simulink model "rotpentemplate"  (R2021b)
settings: Solver=ode45  StartTime=0.0  StopTime=10  RelTol=1e-3  EnableMultiTasking=on
values from neighbouring files (symbols this model uses):
  A = [0 1 0 0 ... (first row only)    [linearize_script.m]    (also in step4_0_linearize_operating_point.m = double(A); step4_linearized_system.mat = [0 0.306815158551 0 -109.913929424 0 1 -60.0152130057 0 126.; syms_test.m = double(A))
  adingain = [adin_gain 1 1 1 1 1]    [hwinit.m]    (also in hwinit_raw.m)
  adinoffs = [adin_offs 0 0 0 0 0]    [hwinit.m]    (also in hwinit_raw.m)
  B = [0 ... (first row only)    [linearize_script.m]    (also in step4_0_linearize_operating_point.m = double(B); step4_linearized_system.mat = [0 0 0 0 858.38566108]; syms_test.m = double(B))
  C = [1 0 0 0 ... (first row only)    [linearize_script.m]    (also in matrixmaker_linearization.m = [b_1_0 - P_3 * theta_d_2 * sin(theta_2)  -P_3 * (theta_d_1 +; step4_0_linearize_operating_point.m = [1 0 0 0 0; step4_linearized_system.mat = [1  0  0  0  0; 0  0  1  0  0]; syms_test.m)
  D = zeros(2,1)    [linearize_script.m]    (also in step4_0_linearize_operating_point.m; step4_linearized_system.mat = [0 0]; syms_test.m)
  daoutgain = 1*[-6]    [hwinit.m]    (also in hwinit_raw.m)
  daoutoffs = [0.00]    [hwinit.m]    (also in hwinit_raw.m)
  h = 0.001    [hwinit.m]    (also in hwinit_raw.m; init_fugi.m = fugiboard('Open', 'Pendulum1'); one_run.m = fugiboard('Open', 'pendulum1'); one_single_run.m = fugiboard('Open', 'pendulum1'))
  K = K1    [step6_1_controller_feedback.m]
  Ke = [165.387583111  -5.89857635124; 3165.93278733  -398.274578992; 81.102554045  215.74157361; 15046.5760039  11054.3649817; 3886.10400765  -704.144825536]    [step5_observor.mat]    (also in step5_observor_design.m = place(A_, B_, 0.5*J)')
  theta_1_0 = pi    (= 3.14159265359)    [hwinit.m]    (also in hwinit_raw.m; step4_0_linearize_operating_point.m; step5_observor_design.m = x_op(1); step6_1_controller_feedback.m = x_op(1))
  theta_2_0 = 0    [hwinit.m]    (also in hwinit_raw.m; step4_0_linearize_operating_point.m; step5_observor_design.m = x_op(3); step6_1_controller_feedback.m = x_op(3))
libraries: slpidlib x2
settings Model: Creator=rbabuska  LastModifiedBy=lyitingli
settings SolverCC: AlgebraicLoopSolver=TrustRegion
settings DataIOCC: LimitDataPoints=on  SaveFormat=Array  ReturnWorkspaceOutputs=off  SignalLoggingName=sigsOut
settings OptimizationCC: BooleanDataType=off  ExpressionDepthLimit=2147483647  InitFltsAndDblsToZero=on  LifeSpan=inf
settings DebuggingCC: SaveWithParameterizedLinksMsg=none  SignalResolutionControl=TryResolveAllWithWarning  MultiTaskDSMMsg=warning  MultiTaskCondExecSysMsg=none  AllowSymbolicDim=off  StateNameClashWarn=warning  SFUnexpectedBacktrackingDiag=warning  SFNoUnconditionalDefaultTransitionDiag=warning  SFExecutionAtInitializationDiag=none  SFMachineParentedDataDiag=warning  ArithmeticOperatorsInVariantConditions=warning
settings HardwareCC: ProdBitPerPointer=32  ProdBitPerSizeT=32  ProdBitPerPtrDiffT=32  ProdLargestAtomicFloat=None  ProdIntDivRoundTo=Undefined  ProdEndianess=Unspecified  ProdWordSize=32  ProdHWDeviceType=32-bit Generic  TargetUnknown=on
settings ModelReferenceCC: PropagateSignalLabelsOutOfModel=off
settings SFSimCC: SimUseLocalCustomCode=off  CustomCodeUndefinedFunction=UseInterfaceOnly
settings RTWCC: RTWUseLocalCustomCode=off
settings CodeAppCC: StateflowObjectComments=on
settings GRTTargetCC: TargetFcnLib=ansi_tfl_tmw.mat  TargetLangStandard=C89/C90 (ANSI)  CombineOutputUpdateFcns=off  GRTInterface=on
settings ConfigComp: CovMetricSettings=dw  CovSaveCumulativeToWorkspaceVar=on  CovSaveSingleToWorkspaceVar=on  CovExternalEMLEnable=off

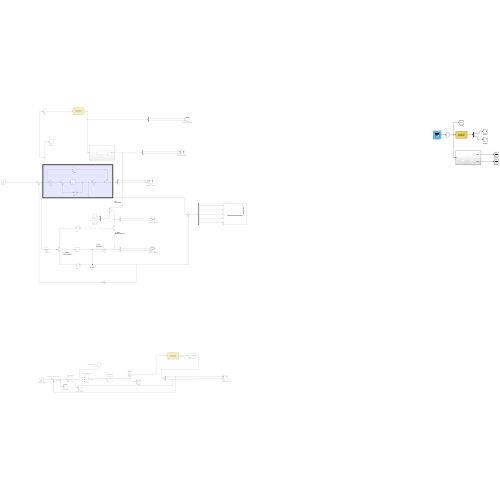
[thumbnail: Simulink's stored preview of the top-level diagram]
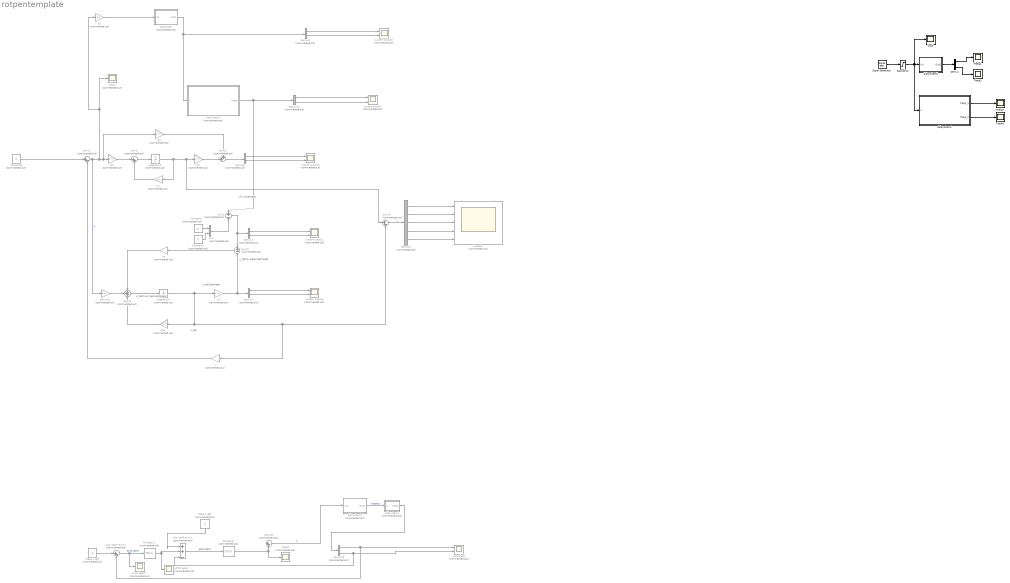
== system rotpentemplate ==
  note: y_hat(k)
      | output estimate
  note: x_hat(k+1)
      | next estimate
  note: y(k)
      | incremetal
  note: x_hat
      | Estimate
  note: x_hat
  A2 : Gain  Commented=on  Gain=A  Multiplication=Matrix(K*u) (u vector)
  B1 : Gain  Commented=on  Gain=-0.1
  B4 : Gain  Commented=on  Gain=B  Multiplication=Matrix(K*u)
  B5 : Gain  Commented=on  Gain=D  Multiplication=Matrix(K*u)
  C3 : Gain  Commented=on  Gain=C  Multiplication=Matrix(K*u) (u vector)
  C4 : Gain  Commented=on  Gain=C  Multiplication=Matrix(K*u) (u vector)
  Constant1 : Constant  Commented=on  Value=pi  SampleTime=-1
  Constant2 : Constant  Commented=on  Value=0  SampleTime=-1
  Constant3 : Constant  Commented=on  Value=0  SampleTime=0.001
  Demux : Demux  Outputs=2
  Demux{1..2,5,7,11,15} (6 alike) : Demux  Commented=on  Outputs=2
  Demux6 : Demux  Commented=on  Outputs=5
  Input : Scope
  Integrator3 : Integrator  Commented=on  InitialCondition=[0; 0; 0; 0; 0]
  Integrator4 : Integrator  Commented=on  InitialCondition=[0; 0; 0; 0; 0]
  Ke : Gain  Commented=on  Gain=Ke  Multiplication=Matrix(K*u) (u vector)
  L : Gain  Commented=on  Gain=1*K  Multiplication=Matrix(K*u) (u vector)
  Mux : Mux  Commented=on  Inputs=2
  PID beam1 : slpidlib/PID Controller  Commented=on  Controller=PID  Form=Parallel  TimeDomain=Continuous-time  UseExternalTs=off  SampleTime=-1  IntegratorMethod=Forward Euler  FilterMethod=Forward Euler  ControllerParametersSource=internal  P=-0.5  I=0  D=-0.02  UseFilter=on  N=100  TunerSelectOption=Transfer Function Based (PID Tuner App)  InitialConditionSource=internal  InitialConditionForIntegrator=0  InitialConditionForFilter=0  DifferentiatorICPrevScaledInput=0  ExternalReset=none  TrackingMode=off  Kt=1  LimitOutput=off  SatLimitsSource=internal  UpperSaturationLimit=inf  LowerSaturationLimit=-inf  LinearizeAsGain=on  AntiWindupMode=none  Kb=1  POutMin=[]  POutMax=[]  IOutMin=[]  IOutMax=[]  DOutMin=[]  DOutMax=[]  NOutMin=[]  NOutMax=[]  SumOutMin=[]  SumOutMax=[]  SaturationOutMin=[]  SaturationOutMax=[]  PParamMin=[]  PParamMax=[]  IParamMin=[]  IParamMax=[]  DParamMin=[]  DParamMax=[]  NParamMin=[]  NParamMax=[]  KbParamMin=[]  KbParamMax=[]  KtParamMin=[]  KtParamMax=[]  KbOutMin=[]  KbOutMax=[]  KtOutMin=[]  KtOutMax=[]  IntegratorOutMin=[]  IntegratorOutMax=[]  FilterOutMin=[]  FilterOutMax=[]  SumI1OutMin=[]  SumI1OutMax=[]  SumI2OutMin=[]  SumI2OutMax=[]  SumI3OutMin=[]  SumI3OutMax=[]  SumI4OutMin=[]  SumI4OutMax=[]  SumDOutMin=[]  SumDOutMax=[]  DifferentiatorOutMin=[]  DifferentiatorOutMax=[]  FilterDiffOutCoefMin=[]  FilterDiffOutCoefMax=[]  ReciprocalOutMin=[]  ReciprocalOutMax=[]  SumDenOutMin=[]  SumDenOutMax=[]  SumNumOutMin=[]  SumNumOutMax=[]  DivideOutMin=[]  DivideOutMax=[]  UdiffTsProdOutMin=[]  UdiffTsProdOutMax=[]  NTsProdOutMin=[]  NTsProdOutMax=[]  UintegralTsProdOutMin=[]  UintegralTsProdOutMax=[]  UngainTsProdOutMin=[]  UngainTsProdOutMax=[]  IntegratorContinuousStateAttributes=''  IntegratorStateMustResolveToSignalObject=off  IntegratorRTWStateStorageClass=Auto  FilterContinuousStateAttributes=''  FilterStateMustResolveToSignalObject=off  FilterRTWStateStorageClass=Auto  ParallelPVariant=InternalParameters  IdealPVariant=Disabled  IVariant=InternalParameters  DVariant=InternalParameters  IntegratorVariant=Continuous  SatVariant=Disabled  AWVariant=Passthrough  PCopyVariant=Disabled  TRVariant=Disabled  FdbkBlocksVariant=Forward  IdealPFdbkVariant=Disabled  SatFdbkVariant=Disabled  DerivativeFilterVariant=ContFilter  NVariant=InternalParameters  NCopyVariant=Disabled  FilterICVariant=InternalICsFilter  IntegratorICVariant=InternalICs  ExternalResetVariant=Disabled  TRSumVariant=Passthrough  SumFdbkVariant=Disabled  SumVariant=Sum_PID  TsampFilterVariant=InternalTs  TsampNgainVariant=Passthrough  TsampIntegralVariant=Passthrough  ExternalSaturationOutDataTypeStr=Inherit: Same as second input
  PID pend1 : slpidlib/PID Controller  Commented=on  Controller=PID  Form=Parallel  TimeDomain=Continuous-time  UseExternalTs=off  SampleTime=-1  IntegratorMethod=Forward Euler  FilterMethod=Forward Euler  ControllerParametersSource=internal  P=-10  I=0  D=-0.01  UseFilter=on  N=100  TunerSelectOption=Transfer Function Based (PID Tuner App)  InitialConditionSource=internal  InitialConditionForIntegrator=0  InitialConditionForFilter=0  DifferentiatorICPrevScaledInput=0  ExternalReset=none  TrackingMode=off  Kt=1  LimitOutput=off  SatLimitsSource=internal  UpperSaturationLimit=inf  LowerSaturationLimit=-inf  LinearizeAsGain=on  AntiWindupMode=none  Kb=1  POutMin=[]  POutMax=[]  IOutMin=[]  IOutMax=[]  DOutMin=[]  DOutMax=[]  NOutMin=[]  NOutMax=[]  SumOutMin=[]  SumOutMax=[]  SaturationOutMin=[]  SaturationOutMax=[]  PParamMin=[]  PParamMax=[]  IParamMin=[]  IParamMax=[]  DParamMin=[]  DParamMax=[]  NParamMin=[]  NParamMax=[]  KbParamMin=[]  KbParamMax=[]  KtParamMin=[]  KtParamMax=[]  KbOutMin=[]  KbOutMax=[]  KtOutMin=[]  KtOutMax=[]  IntegratorOutMin=[]  IntegratorOutMax=[]  FilterOutMin=[]  FilterOutMax=[]  SumI1OutMin=[]  SumI1OutMax=[]  SumI2OutMin=[]  SumI2OutMax=[]  SumI3OutMin=[]  SumI3OutMax=[]  SumI4OutMin=[]  SumI4OutMax=[]  SumDOutMin=[]  SumDOutMax=[]  DifferentiatorOutMin=[]  DifferentiatorOutMax=[]  FilterDiffOutCoefMin=[]  FilterDiffOutCoefMax=[]  ReciprocalOutMin=[]  ReciprocalOutMax=[]  SumDenOutMin=[]  SumDenOutMax=[]  SumNumOutMin=[]  SumNumOutMax=[]  DivideOutMin=[]  DivideOutMax=[]  UdiffTsProdOutMin=[]  UdiffTsProdOutMax=[]  NTsProdOutMin=[]  NTsProdOutMax=[]  UintegralTsProdOutMin=[]  UintegralTsProdOutMax=[]  UngainTsProdOutMin=[]  UngainTsProdOutMax=[]  IntegratorContinuousStateAttributes=''  IntegratorStateMustResolveToSignalObject=off  IntegratorRTWStateStorageClass=Auto  FilterContinuousStateAttributes=''  FilterStateMustResolveToSignalObject=off  FilterRTWStateStorageClass=Auto  ParallelPVariant=InternalParameters  IdealPVariant=Disabled  IVariant=InternalParameters  DVariant=InternalParameters  IntegratorVariant=Continuous  SatVariant=Disabled  AWVariant=Passthrough  PCopyVariant=Disabled  TRVariant=Disabled  FdbkBlocksVariant=Forward  IdealPFdbkVariant=Disabled  SatFdbkVariant=Disabled  DerivativeFilterVariant=ContFilter  NVariant=InternalParameters  NCopyVariant=Disabled  FilterICVariant=InternalICsFilter  IntegratorICVariant=InternalICs  ExternalResetVariant=Disabled  TRSumVariant=Passthrough  SumFdbkVariant=Disabled  SumVariant=Sum_PID  TsampFilterVariant=InternalTs  TsampNgainVariant=Passthrough  TsampIntegralVariant=Passthrough  ExternalSaturationOutDataTypeStr=Inherit: Same as second input
  Saturation : Saturate  UpperLimit=1  LowerLimit=-1
  Scope1 : Scope  Commented=on  NumInputPorts=5
  Signal Generator : SignalGenerator  Amplitude=0.3*0.5  Frequency=[1 2]
  Subsystem : Subsystem  Commented=on
      mask Display: disp('Rotational\nPendulum')
  Subsystem1 : Subsystem  Commented=on
  Subsystem2 : Subsystem  Commented=on
  Subsystem3 : Subsystem  Commented=on
      mask Display: disp('Rotational\nPendulum')
  Subsystem4 : Subsystem
  Subsystem5 : Subsystem
      mask Display: disp('Rotational\nPendulum')
  Sum beam error1 : Sum  Commented=on  Inputs=|+-
  Sum pend error1 : Sum  Commented=on  Inputs=|++-
  Sum1 : Sum  Commented=on  Inputs=+|-
  Sum10 : Sum  Commented=on  Inputs=++|
  Sum11 : Sum  Commented=on  Inputs=|+-
  Sum12 : Sum  Commented=on  Inputs=+|-
  Sum13 : Sum  Commented=on  Inputs=+++
  Sum14 : Sum  Commented=on  Inputs=|+-
  Sum9 : Sum  Commented=on  Inputs=|++
  Theta 1 ref2 : Constant  Commented=on  Value=pi
  Theta 2 ref2 : Constant  Commented=on  Value=0
  Theta{1..4} (4 alike) : Scope
  controled1 : Scope  Commented=on  NumInputPorts=2
  disturb1 : Sum  Commented=on  Inputs=|++
  error beam1 : Scope  Commented=on
  gamma1 : Gain  Commented=on  Gain=B  Multiplication=Matrix(K*u)
  input4 : Scope  Commented=on
  input8 : Scope  Commented=on
  phi1 : Gain  Commented=on  Gain=A  Multiplication=Matrix(K*u) (u vector)
  ref for pend1 : Scope  Commented=on
  system output{1..4,7} (5 alike) : Scope  Commented=on  NumInputPorts=2
  wires:
  Sum14/1 -> Demux6/1  "u"
  Constant3/1 -> Sum11/1
  Sum12/1 -> Ke/1
  Sum10/1 -> Demux5/1
  Integrator3/1 -> C3/1, Sum14/1, A2/1
  Sum9/1 -> Integrator3/1
  Demux7/1 -> system output4/1
  Demux5/2 -> system output3/2
  Ke/1 -> Sum13/1
  L/1 -> Sum11/2
  B4/1 -> Sum9/1
  phi1/1 -> Sum13/3
  Demux5/1 -> system output3/1
  Demux6/3 -> Scope1/3
  Demux7/2 -> system output4/2
  Demux6/5 -> Scope1/5
  B5/1 -> Sum10/1
  A2/1 -> Sum9/2
  Demux6/4 -> Scope1/4
  Sum13/1 -> Integrator4/1
  C4/1 -> Sum12/2, Demux7/1
  Demux11/2 -> system output7/2
  Demux6/1 -> Scope1/1
  Integrator4/1 -> phi1/1, L/1, Sum14/2, C4/1
  gamma1/1 -> Sum13/2
  Sum11/1 -> B1/1, input4/1, B4/1, B5/1, gamma1/1  "u"
  C3/1 -> Sum10/2
  Demux11/1 -> system output7/1
  Demux6/2 -> Scope1/2
  Sum1/1 -> Demux1/1, Sum12/1
  Constant1/1 -> Mux/1
  Constant2/1 -> Mux/2
  Demux1/1 -> system output1/1
  Demux1/2 -> system output1/2
  Mux/1 -> Sum1/2
  Subsystem2/1(theta) -> Sum1/1, Demux11/1
  Demux2/2 -> system output2/2
  Demux2/1 -> system output2/1
  Subsystem/1(Out1) -> Demux2/1, Subsystem2/1(u)
  B1/1 -> Subsystem/1(In1)
  Demux15/1 -> controled1/1, Sum beam error1/2
  Sum beam error1/1 -> PID beam1/1, error beam1/1  "error term"
  disturb1/1 -> Subsystem3/1(In1)  "u"
  Theta 2 ref2/1 -> Sum pend error1/1
  Theta 1 ref2/1 -> Sum beam error1/1
  Demux15/2 -> Sum pend error1/3, controled1/2
  Sum pend error1/1 -> PID pend1/1  "error term"
  PID beam1/1 -> ref for pend1/1, Sum pend error1/2
  PID pend1/1 -> input8/1, disturb1/2
  Subsystem3/1(Out1) -> Subsystem1/1(u)  "output y"
  Subsystem1/1(theta) -> Demux15/1
  Demux/1 -> Theta1/1
  Subsystem5/1(Out1) -> Demux/1
  Demux/2 -> Theta2/1
  Signal Generator/1 -> Saturation/1
  Saturation/1 -> Subsystem4/1(u), Subsystem5/1(In1), Input/1
  Subsystem4/1(theta_1) -> Theta3/1
  Subsystem4/2(theta_2) -> Theta4/1

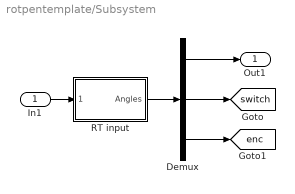
== system rotpentemplate/Subsystem ==
  In1 : Inport
  Demux : Demux  Outputs=[2 4 1]
  RT input : Subsystem  mask{Ts=h, channels=[6 7]}
      mask prompts: Ts "Sample time [s]:"; channels "Channels to read (e.g., [6 7])"
      mask init:
      | hwinit;
      | 
      | % initialize FPGA
      | fugihandle = fugiboard('Open', 'Pendulum1');
      | fugihandle.WatchdogTimeout = 0.5;
      | fugiboard('SetParams', fugihandle);
      | fugiboard('Write', fugihandle, 0, 0, 0, 0);  % dummy write to sync interface board
      | fugiboard('Write', fugihandle, 5, 1, 0, 0);  % reset position, activate relay
      | data = fugiboard('Read', fugihandle);        % get version info from FPGA
      | % model = bitshift(data(1), -5); 
      | % version = bitand(data(1), 31);
      | % disp(sprintf('FPGA setup %d, version %d', model, version)); % for the B&P it should say 1 1, or else there is a problem
      | fugiboard('Write', fugihandle, 0, 1, 0, 0);  % end reset
      | pause(0.1);                         % give relay some time to respond
      mask Display: disp('Rotational\nPendulum')
  Out1 : Outport
  tag scope: enc=global, switch=global
  wires:
  RT input/1(Angles) -> Demux/1
  Demux/1 -> Out1/1
  Demux/2 -> [switch]
  Demux/3 -> [enc]
  In1/1 -> RT input/1(Motors)

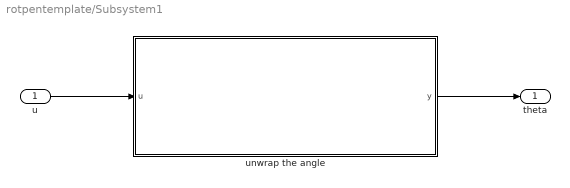
== system rotpentemplate/Subsystem1 ==
  u : Inport
  unwrap the angle : MATLAB Function  TreatAsAtomicUnit=on
  theta : Outport
  wires:
  u/1 -> unwrap the angle/1(u)
  unwrap the angle/1(y) -> theta/1

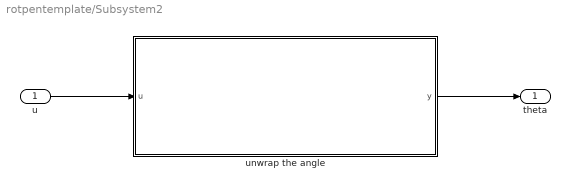
== system rotpentemplate/Subsystem2 ==
  u : Inport
  unwrap the angle : MATLAB Function  TreatAsAtomicUnit=on
  theta : Outport
  wires:
  u/1 -> unwrap the angle/1(u)
  unwrap the angle/1(y) -> theta/1

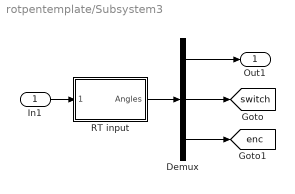
== system rotpentemplate/Subsystem3 ==
  In1 : Inport
  Demux : Demux  Outputs=[2 4 1]
  RT input : Subsystem  mask{Ts=h, channels=[6 7]}
      mask prompts: Ts "Sample time [s]:"; channels "Channels to read (e.g., [6 7])"
      mask init: same as rotpentemplate/Subsystem/RT input
      mask Display: disp('Rotational\nPendulum')
  Out1 : Outport
  tag scope: enc=global, switch=global
  wires:
  RT input/1(Angles) -> Demux/1
  Demux/1 -> Out1/1
  Demux/2 -> [switch]
  Demux/3 -> [enc]
  In1/1 -> RT input/1(Motors)

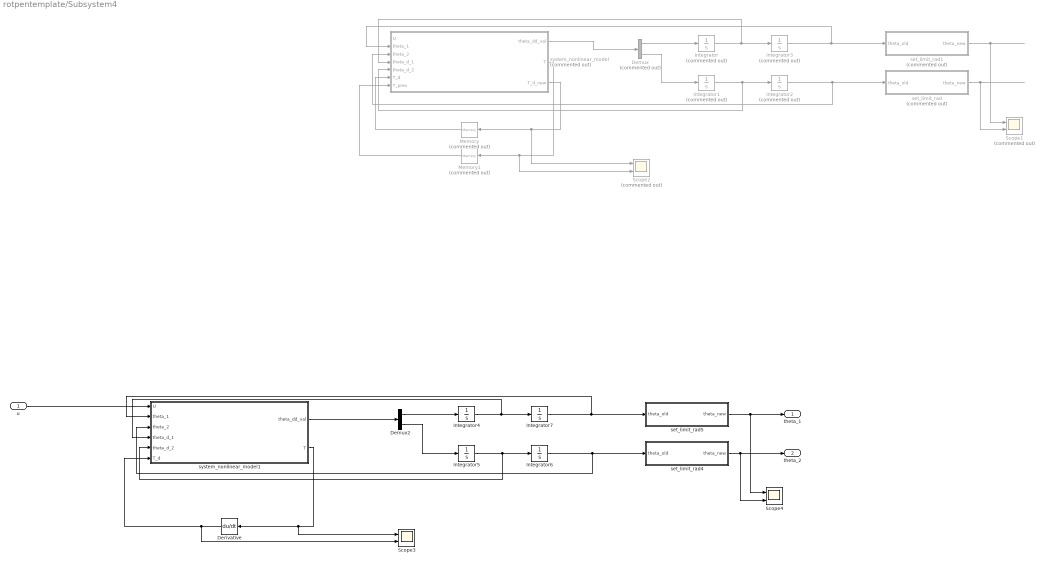
== system rotpentemplate/Subsystem4 ==
  u : Inport
  Demux : Demux  Commented=on  Outputs=2
  Demux2 : Demux  Outputs=2
  Derivative : Derivative  CoefficientInTFapproximation=0
  Integrator : Integrator  Commented=on
  Integrator1 : Integrator  Commented=on
  Integrator2 : Integrator  Commented=on  InitialCondition=theta_2_0
  Integrator3 : Integrator  Commented=on  InitialCondition=theta_1_0
  Integrator4 : Integrator
  Integrator5 : Integrator
  Integrator6 : Integrator  InitialCondition=theta_2_0
  Integrator7 : Integrator  InitialCondition=theta_1_0
  Memory : Memory  Commented=on  InheritSampleTime=on
  Memory1 : Memory  Commented=on  InheritSampleTime=on
  Scope1 : Scope  Commented=on  NumInputPorts=2
  Scope2 : Scope  Commented=on  NumInputPorts=2
  Scope3 : Scope  NumInputPorts=2
  Scope4 : Scope  NumInputPorts=2
  set_limit_rad : MATLAB Function  Commented=on  TreatAsAtomicUnit=on
  set_limit_rad1 : MATLAB Function  Commented=on  TreatAsAtomicUnit=on
  set_limit_rad4 : MATLAB Function  TreatAsAtomicUnit=on
  set_limit_rad5 : MATLAB Function  TreatAsAtomicUnit=on
  system_nonlinear_model : MATLAB Function  Commented=on  TreatAsAtomicUnit=on
  system_nonlinear_model1 : MATLAB Function  TreatAsAtomicUnit=on
  theta_1 : Outport
  theta_2 : Outport  Port=2
  wires:
  Derivative/1 -> Scope3/2, system_nonlinear_model1/6(T_d)
  system_nonlinear_model1/2(T) -> Scope3/1, Derivative/1
  set_limit_rad4/1(theta_new) -> theta_2/1, Scope4/2
  Integrator4/1 -> system_nonlinear_model1/4(theta_d_1), Integrator7/1
  system_nonlinear_model1/1(theta_dd_val) -> Demux2/1
  Integrator6/1 -> system_nonlinear_model1/3(theta_2), set_limit_rad4/1(theta_old)
  u/1 -> system_nonlinear_model1/1(U)
  Integrator7/1 -> set_limit_rad5/1(theta_old), system_nonlinear_model1/2(theta_1)
  Integrator5/1 -> system_nonlinear_model1/5(theta_d_2), Integrator6/1
  Demux2/1 -> Integrator4/1
  Demux2/2 -> Integrator5/1
  set_limit_rad5/1(theta_new) -> theta_1/1, Scope4/1
  system_nonlinear_model/2(T) -> Scope2/2, Memory1/1
  Demux/1 -> Integrator/1
  Integrator/1 -> system_nonlinear_model/4(theta_d_1), Integrator3/1
  Demux/2 -> Integrator1/1
  Integrator3/1 -> set_limit_rad1/1(theta_old), system_nonlinear_model/2(theta_1)
  system_nonlinear_model/1(theta_dd_val) -> Demux/1
  set_limit_rad/1(theta_new) -> Scope1/2
  Integrator1/1 -> system_nonlinear_model/5(theta_d_2), Integrator2/1
  system_nonlinear_model/3(T_d_new) -> Scope2/1, Memory/1
  Integrator2/1 -> system_nonlinear_model/3(theta_2), set_limit_rad/1(theta_old)
  Memory/1 -> system_nonlinear_model/6(T_d)
  ? -> system_nonlinear_model/1(U)
  set_limit_rad1/1(theta_new) -> Scope1/1
  Memory1/1 -> system_nonlinear_model/7(T_prev)

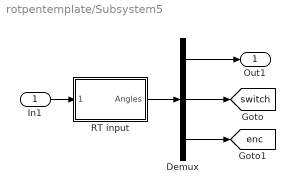
== system rotpentemplate/Subsystem5 ==
  In1 : Inport
  Demux : Demux  Outputs=[2 4 1]
  RT input : Subsystem  mask{Ts=h, channels=[6 7]}
      mask prompts: Ts "Sample time [s]:"; channels "Channels to read (e.g., [6 7])"
      mask init: same as rotpentemplate/Subsystem/RT input
      mask Display: disp('Rotational\nPendulum')
  Out1 : Outport
  tag scope: enc=global, switch=global
  wires:
  RT input/1(Angles) -> Demux/1
  Demux/1 -> Out1/1
  Demux/2 -> [switch]
  Demux/3 -> [enc]
  In1/1 -> RT input/1(Motors)

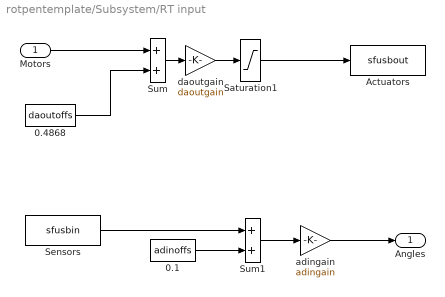
== system rotpentemplate/Subsystem/RT input ==
  Motors : Inport
  0.1 : Constant  Value=adinoffs
  0.4868 : Constant  Value=daoutoffs
  Actuators : S-Function  FunctionName=sfusbout  Parameters=Ts, fugihandle  SFunctionDeploymentMode=off  EnableBusSupport=off
  Saturation1 : Saturate  UpperLimit=10  LowerLimit=-10
  Sensors : S-Function  FunctionName=sfusbin  Parameters=Ts, fugihandle, channels  SFunctionDeploymentMode=off  EnableBusSupport=off
  Sum : Sum  InputSameDT=on  SaturateOnIntegerOverflow=on  OutDataTypeStr=Inherit: Same as first input
  Sum1 : Sum  InputSameDT=on  SaturateOnIntegerOverflow=on  OutDataTypeStr=Inherit: Same as first input
  adingain : Gain  Gain=adingain  SaturateOnIntegerOverflow=on  OutDataTypeStr=Inherit: Same as input  ParamDataTypeStr=Inherit: Same as input
  daoutgain : Gain  Gain=daoutgain  SaturateOnIntegerOverflow=on  OutDataTypeStr=Inherit: Same as input  ParamDataTypeStr=Inherit: Same as input
  Angles : Outport
  wires:
  Sum/1 -> daoutgain/1
  0.4868/1 -> Sum/2
  Motors/1 -> Sum/1
  Sum1/1 -> adingain/1
  0.1/1 -> Sum1/2
  adingain/1 -> Angles/1
  Saturation1/1 -> Actuators/1
  daoutgain/1 -> Saturation1/1
  Sensors/1 -> Sum1/1

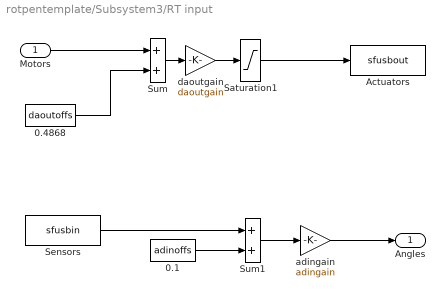
== system rotpentemplate/Subsystem3/RT input ==
  Motors : Inport
  0.1 : Constant  Value=adinoffs
  0.4868 : Constant  Value=daoutoffs
  Actuators : S-Function  FunctionName=sfusbout  Parameters=Ts, fugihandle  SFunctionDeploymentMode=off  EnableBusSupport=off
  Saturation1 : Saturate  UpperLimit=10  LowerLimit=-10
  Sensors : S-Function  FunctionName=sfusbin  Parameters=Ts, fugihandle, channels  SFunctionDeploymentMode=off  EnableBusSupport=off
  Sum : Sum  InputSameDT=on  SaturateOnIntegerOverflow=on  OutDataTypeStr=Inherit: Same as first input
  Sum1 : Sum  InputSameDT=on  SaturateOnIntegerOverflow=on  OutDataTypeStr=Inherit: Same as first input
  adingain : Gain  Gain=adingain  SaturateOnIntegerOverflow=on  OutDataTypeStr=Inherit: Same as input  ParamDataTypeStr=Inherit: Same as input
  daoutgain : Gain  Gain=daoutgain  SaturateOnIntegerOverflow=on  OutDataTypeStr=Inherit: Same as input  ParamDataTypeStr=Inherit: Same as input
  Angles : Outport
  wires:
  Sum/1 -> daoutgain/1
  0.4868/1 -> Sum/2
  Motors/1 -> Sum/1
  Sum1/1 -> adingain/1
  0.1/1 -> Sum1/2
  adingain/1 -> Angles/1
  Saturation1/1 -> Actuators/1
  daoutgain/1 -> Saturation1/1
  Sensors/1 -> Sum1/1

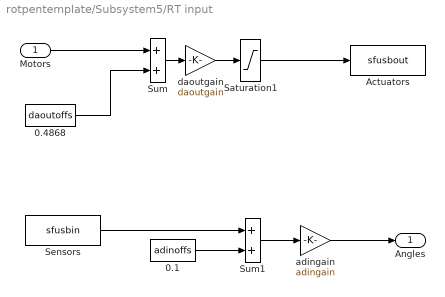
== system rotpentemplate/Subsystem5/RT input ==
  Motors : Inport
  0.1 : Constant  Value=adinoffs
  0.4868 : Constant  Value=daoutoffs
  Actuators : S-Function  FunctionName=sfusbout  Parameters=Ts, fugihandle  SFunctionDeploymentMode=off  EnableBusSupport=off
  Saturation1 : Saturate  UpperLimit=10  LowerLimit=-10
  Sensors : S-Function  FunctionName=sfusbin  Parameters=Ts, fugihandle, channels  SFunctionDeploymentMode=off  EnableBusSupport=off
  Sum : Sum  InputSameDT=on  SaturateOnIntegerOverflow=on  OutDataTypeStr=Inherit: Same as first input
  Sum1 : Sum  InputSameDT=on  SaturateOnIntegerOverflow=on  OutDataTypeStr=Inherit: Same as first input
  adingain : Gain  Gain=adingain  SaturateOnIntegerOverflow=on  OutDataTypeStr=Inherit: Same as input  ParamDataTypeStr=Inherit: Same as input
  daoutgain : Gain  Gain=daoutgain  SaturateOnIntegerOverflow=on  OutDataTypeStr=Inherit: Same as input  ParamDataTypeStr=Inherit: Same as input
  Angles : Outport
  wires:
  Sum/1 -> daoutgain/1
  0.4868/1 -> Sum/2
  Motors/1 -> Sum/1
  Sum1/1 -> adingain/1
  0.1/1 -> Sum1/2
  adingain/1 -> Angles/1
  Saturation1/1 -> Actuators/1
  daoutgain/1 -> Saturation1/1
  Sensors/1 -> Sum1/1

== matlab function rotpentemplate/Subsystem1/unwrap the angle ==
  settings: updateMethod=DISCRETE  sampleTime=0.001
  data: u input size=2; y output size=2
function y = unwrap_angle(u)

y = unwrap(u);
% y = u;

== matlab function rotpentemplate/Subsystem4/set_limit_rad ==
  settings: updateMethod=DISCRETE  sampleTime=0.001
  data: theta_old input size=1; theta_new output size=1
function theta_new   = set_limit_rad(theta_old)

theta_new = theta_old - floor(theta_old / 2 / pi) * 2 * pi;
theta_new = theta_old;

== matlab function rotpentemplate/Subsystem4/set_limit_rad1 ==
  settings: updateMethod=DISCRETE  sampleTime=0.001
  data: theta_old input size=1; theta_new output size=1
function theta_new   = set_limit_rad(theta_old)

theta_new = theta_old - floor(theta_old / 2 / pi) * 2 * pi;
theta_new = theta_old;

== matlab function rotpentemplate/Subsystem4/system_nonlinear_model1 ==
  settings: updateMethod=DISCRETE  sampleTime=0.001
  data: U input size=1; theta_dd_val output size=2; T output; theta_1 input size=1; theta_2 input size=1; theta_d_1 input size=1; theta_d_2 input size=1; T_d input
function [theta_dd_val, T]   = get_theta_dt_dt(U, theta_1, theta_2, theta_d_1, theta_d_2, T_d)


u = U(1);
k_m_0 = 25.9;
tau_e_0 = 0.03;

T = k_m_0 * u - tau_e_0 * T_d;






theta_dd_val = [
                                                                                                                                                                   (2177205792337185200000*sin(theta_1 + theta_2)*(7101996468378179*cos(theta_2) + 5837472162125388))/(59390441777463697512*cos(theta_2) + 157619855740175396464645510487628125*cos(theta_2)^2 - 67469767625708245300871903596602750000) - theta_d_2*((1152921504606846976*(7101996468378179*cos(theta_2) + 5837472162125388))/(59390441777463697512*cos(theta_2) + 157619855740175396464645510487628125*cos(theta_2)^2 - 67469767625708245300871903596602750000) + (336507359412909324930676272031334400000*sin(theta_2)*((7101996468378179*theta_d_1)/18446744073709551616 + (7101996468378179*theta_d_2)/18446744073709551616))/(59390441777463697512*cos(theta_2) + 157619855740175396464645510487628125*cos(theta_2)^2 - 67469767625708245300871903596602750000)) - theta_d_1*((336507359412909324930676272031334400000*((7101996468378179*theta_d_2*sin(theta_2))/18446744073709551616 - 5171/250))/(59390441777463697512*cos(theta_2) + 157619855740175396464645510487628125*cos(theta_2)^2 - 67469767625708245300871903596602750000) + (22193738963681809375*theta_d_1*sin(theta_2)*(7101996468378179*cos(theta_2) + 5837472162125388))/(59390441777463697512*cos(theta_2) + 157619855740175396464645510487628125*cos(theta_2)^2 - 67469767625708245300871903596602750000)) - (336507359412909324930676272031334400000*T)/(59390441777463697512*cos(theta_2) + 157619855740175396464645510487628125*cos(theta_2)^2 - 67469767625708245300871903596602750000) - (336507359412909324930676272031334400000*((5443014480842963*sin(theta_1 + theta_2))/144115188075855872 + (3446064362871357*sin(theta_1))/72057594037927936))/(59390441777463697512*cos(theta_2) + 157619855740175396464645510487628125*cos(theta_2)^2 - 67469767625708245300871903596602750000);
theta_d_1*((57646075230342348800000*(7101996468378179*cos(theta_2) + 5837472162125388)*((7101996468378179*theta_d_2*sin(theta_2))/18446744073709551616 - 5171/250))/(59390441777463697512*cos(theta_2) + 157619855740175396464645510487628125*cos(theta_2)^2 - 67469767625708245300871903596602750000) + (7272444383619255296*theta_d_1*sin(theta_2)*(43347146413441024*cos(theta_2) + 11304968154247740625))/(59390441777463697512*cos(theta_2) + 157619855740175396464645510487628125*cos(theta_2)^2 - 67469767625708245300871903596602750000)) + theta_d_2*((1180591620717411303424*(43347146413441024*cos(theta_2) + 11304968154247740625))/(3125*(59390441777463697512*cos(theta_2) + 157619855740175396464645510487628125*cos(theta_2)^2 - 67469767625708245300871903596602750000)) + (57646075230342348800000*sin(theta_2)*(7101996468378179*cos(theta_2) + 5837472162125388)*((7101996468378179*theta_d_1)/18446744073709551616 + (7101996468378179*theta_d_2)/18446744073709551616))/(59390441777463697512*cos(theta_2) + 157619855740175396464645510487628125*cos(theta_2)^2 - 67469767625708245300871903596602750000)) + (57646075230342348800000*T*(7101996468378179*cos(theta_2) + 5837472162125388))/(59390441777463697512*cos(theta_2) + 157619855740175396464645510487628125*cos(theta_2)^2 - 67469767625708245300871903596602750000) + (57646075230342348800000*(7101996468378179*cos(theta_2) + 5837472162125388)*((5443014480842963*sin(theta_1 + theta_2))/144115188075855872 + (3446064362871357*sin(theta_1))/72057594037927936))/(59390441777463697512*cos(theta_2) + 157619855740175396464645510487628125*cos(theta_2)^2 - 67469767625708245300871903596602750000) - (713426794033048846336*sin(theta_1 + theta_2)*(43347146413441024*cos(theta_2) + 11304968154247740625))/(59390441777463697512*cos(theta_2) + 157619855740175396464645510487628125*cos(theta_2)^2 - 67469767625708245300871903596602750000)     
];

== matlab function rotpentemplate/Subsystem4/system_nonlinear_model ==
  settings: updateMethod=DISCRETE  sampleTime=0.001
  data: U input size=1; theta_dd_val output size=2; T output; theta_1 input size=1; theta_2 input size=1; theta_d_1 input size=1; theta_d_2 input size=1; T_d input; T_prev input; T_d_new output
function [theta_dd_val, T, T_d_new]   = get_theta_dt_dt(U, theta_1, theta_2, theta_d_1, theta_d_2, T_d, T_prev)


u = U(1);
k_m_0 = 15;
tau_e_0 = 0.03;

T = k_m_0 * u - tau_e_0 * T_d;



theta_dd_val = [
                                                                                                                                                                   (2177205792337185200000*sin(theta_1 + theta_2)*(7101996468378179*cos(theta_2) + 5837472162125388))/(59390441777463697512*cos(theta_2) + 157619855740175396464645510487628125*cos(theta_2)^2 - 67469767625708245300871903596602750000) - theta_d_2*((1152921504606846976*(7101996468378179*cos(theta_2) + 5837472162125388))/(59390441777463697512*cos(theta_2) + 157619855740175396464645510487628125*cos(theta_2)^2 - 67469767625708245300871903596602750000) + (336507359412909324930676272031334400000*sin(theta_2)*((7101996468378179*theta_d_1)/18446744073709551616 + (7101996468378179*theta_d_2)/18446744073709551616))/(59390441777463697512*cos(theta_2) + 157619855740175396464645510487628125*cos(theta_2)^2 - 67469767625708245300871903596602750000)) - theta_d_1*((336507359412909324930676272031334400000*((7101996468378179*theta_d_2*sin(theta_2))/18446744073709551616 - 5171/250))/(59390441777463697512*cos(theta_2) + 157619855740175396464645510487628125*cos(theta_2)^2 - 67469767625708245300871903596602750000) + (22193738963681809375*theta_d_1*sin(theta_2)*(7101996468378179*cos(theta_2) + 5837472162125388))/(59390441777463697512*cos(theta_2) + 157619855740175396464645510487628125*cos(theta_2)^2 - 67469767625708245300871903596602750000)) - (336507359412909324930676272031334400000*T)/(59390441777463697512*cos(theta_2) + 157619855740175396464645510487628125*cos(theta_2)^2 - 67469767625708245300871903596602750000) - (336507359412909324930676272031334400000*((5443014480842963*sin(theta_1 + theta_2))/144115188075855872 + (3446064362871357*sin(theta_1))/72057594037927936))/(59390441777463697512*cos(theta_2) + 157619855740175396464645510487628125*cos(theta_2)^2 - 67469767625708245300871903596602750000);
theta_d_1*((57646075230342348800000*(7101996468378179*cos(theta_2) + 5837472162125388)*((7101996468378179*theta_d_2*sin(theta_2))/18446744073709551616 - 5171/250))/(59390441777463697512*cos(theta_2) + 157619855740175396464645510487628125*cos(theta_2)^2 - 67469767625708245300871903596602750000) + (7272444383619255296*theta_d_1*sin(theta_2)*(43347146413441024*cos(theta_2) + 11304968154247740625))/(59390441777463697512*cos(theta_2) + 157619855740175396464645510487628125*cos(theta_2)^2 - 67469767625708245300871903596602750000)) + theta_d_2*((1180591620717411303424*(43347146413441024*cos(theta_2) + 11304968154247740625))/(3125*(59390441777463697512*cos(theta_2) + 157619855740175396464645510487628125*cos(theta_2)^2 - 67469767625708245300871903596602750000)) + (57646075230342348800000*sin(theta_2)*(7101996468378179*cos(theta_2) + 5837472162125388)*((7101996468378179*theta_d_1)/18446744073709551616 + (7101996468378179*theta_d_2)/18446744073709551616))/(59390441777463697512*cos(theta_2) + 157619855740175396464645510487628125*cos(theta_2)^2 - 67469767625708245300871903596602750000)) + (57646075230342348800000*T*(7101996468378179*cos(theta_2) + 5837472162125388))/(59390441777463697512*cos(theta_2) + 157619855740175396464645510487628125*cos(theta_2)^2 - 67469767625708245300871903596602750000) + (57646075230342348800000*(7101996468378179*cos(theta_2) + 5837472162125388)*((5443014480842963*sin(theta_1 + theta_2))/144115188075855872 + (3446064362871357*sin(theta_1))/72057594037927936))/(59390441777463697512*cos(theta_2) + 157619855740175396464645510487628125*cos(theta_2)^2 - 67469767625708245300871903596602750000) - (713426794033048846336*sin(theta_1 + theta_2)*(43347146413441024*cos(theta_2) + 11304968154247740625))/(59390441777463697512*cos(theta_2) + 157619855740175396464645510487628125*cos(theta_2)^2 - 67469767625708245300871903596602750000)];
 
%                                                                                                        (50632000000*((3*T_d)/100 - 15*u))/(7*(3388000*cos(theta_2)^2 - 1450246047)) - theta_d_2*((160*(7700*cos(theta_2) + 6329))/(7*(3388000*cos(theta_2)^2 - 1450246047)) + (50632000000*sin(theta_2)*((77*theta_d_1)/200000 + (77*theta_d_2)/200000))/(7*(3388000*cos(theta_2)^2 - 1450246047))) - (50632000000*((75537*sin(theta_1 + theta_2))/2000000 + (38259*sin(theta_1))/800000))/(7*(3388000*cos(theta_2)^2 - 1450246047)) - theta_d_1*((50632000000*((77*theta_d_2*sin(theta_2))/200000 - 5171/250))/(7*(3388000*cos(theta_2)^2 - 1450246047)) + (440*theta_d_1*sin(theta_2)*(7700*cos(theta_2) + 6329))/(3388000*cos(theta_2)^2 - 1450246047)) + (43164*sin(theta_1 + theta_2)*(7700*cos(theta_2) + 6329))/(3388000*cos(theta_2)^2 - 1450246047);
% theta_d_2*((80*(30800*cos(theta_2) + 8032663))/(7*(3388000*cos(theta_2)^2 - 1450246047)) + (8000000*sin(theta_2)*((77*theta_d_1)/200000 + (77*theta_d_2)/200000)*(7700*cos(theta_2) + 6329))/(7*(3388000*cos(theta_2)^2 - 1450246047))) + theta_d_1*((8000000*((77*theta_d_2*sin(theta_2))/200000 - 5171/250)*(7700*cos(theta_2) + 6329))/(7*(3388000*cos(theta_2)^2 - 1450246047)) + (220*theta_d_1*sin(theta_2)*(30800*cos(theta_2) + 8032663))/(3388000*cos(theta_2)^2 - 1450246047)) - (21582*sin(theta_1 + theta_2)*(30800*cos(theta_2) + 8032663))/(3388000*cos(theta_2)^2 - 1450246047) + (8000000*(7700*cos(theta_2) + 6329)*((75537*sin(theta_1 + theta_2))/2000000 + (38259*sin(theta_1))/800000))/(7*(3388000*cos(theta_2)^2 - 1450246047)) - (8000000*(7700*cos(theta_2) + 6329)*((3*T_d)/100 - 15*u))/(7*(3388000*cos(theta_2)^2 - 1450246047))];
%  
%                                                                                                         (43164*sin(theta_1 + theta_2)*(7700*cos(theta_2) + 6329))/(3388000*cos(theta_2)^2 - 1450246047) - (759480000000*u)/(7*(3388000*cos(theta_2)^2 - 1450246047)) - theta_d_2*((160*(7700*cos(theta_2) + 6329))/(7*(3388000*cos(theta_2)^2 - 1450246047)) + (50632000000*sin(theta_2)*((77*theta_d_1)/200000 + (77*theta_d_2)/200000))/(7*(3388000*cos(theta_2)^2 - 1450246047))) - (50632000000*((75537*sin(theta_1 + theta_2))/2000000 + (38259*sin(theta_1))/800000))/(7*(3388000*cos(theta_2)^2 - 1450246047)) - theta_d_1*((50632000000*((77*theta_d_2*sin(theta_2))/200000 - 5171/250))/(7*(3388000*cos(theta_2)^2 - 1450246047)) + (440*theta_d_1*sin(theta_2)*(7700*cos(theta_2) + 6329))/(3388000*cos(theta_2)^2 - 1450246047))
% theta_d_2*((80*(30800*cos(theta_2) + 8032663))/(7*(3388000*cos(theta_2)^2 - 1450246047)) + (8000000*sin(theta_2)*((77*theta_d_1)/200000 + (77*theta_d_2)/200000)*(7700*cos(theta_2) + 6329))/(7*(3388000*cos(theta_2)^2 - 1450246047))) + theta_d_1*((8000000*((77*theta_d_2*sin(theta_2))/200000 - 5171/250)*(7700*cos(theta_2) + 6329))/(7*(3388000*cos(theta_2)^2 - 1450246047)) + (220*theta_d_1*sin(theta_2)*(30800*cos(theta_2) + 8032663))/(3388000*cos(theta_2)^2 - 1450246047)) + (120000000*u*(7700*cos(theta_2) + 6329))/(7*(3388000*cos(theta_2)^2 - 1450246047)) - (21582*sin(theta_1 + theta_2)*(30800*cos(theta_2) + 8032663))/(3388000*cos(theta_2)^2 - 1450246047) + (8000000*(7700*cos(theta_2) + 6329)*((75537*sin(theta_1 + theta_2))/2000000 + (38259*sin(theta_1))/800000))/(7*(3388000*cos(theta_2)^2 - 1450246047))
%  

T_d_new = (T - T_prev)/1;

== matlab function rotpentemplate/Subsystem4/set_limit_rad4 ==
  settings: updateMethod=DISCRETE  sampleTime=0.001
  data: theta_old input size=1; theta_new output size=1
function theta_new   = set_limit_rad(theta_old)

% theta_new = theta_old - floor(theta_old / 2 / pi) * 2 * pi;
theta_new = theta_old;

== matlab function rotpentemplate/Subsystem4/set_limit_rad5 ==
  settings: updateMethod=DISCRETE  sampleTime=0.001
  data: theta_old input size=1; theta_new output size=1
function theta_new   = set_limit_rad(theta_old)

% theta_new = theta_old - floor(theta_old / 2 / pi) * 2 * pi;
theta_new = theta_old;

== matlab function rotpentemplate/Subsystem2/unwrap the angle ==
  settings: updateMethod=DISCRETE  sampleTime=0.001
  data: u input size=2; y output size=2
function y = unwrap_angle(u)

y = unwrap(u);
% y = u;
